simulink model "networked"  (Simulink 4.00)
settings: Solver=ode45  StartTime=0.0  StopTime=2  RelTol=1e-3
libraries: truetime x7
settings Model: Creator=anton  LastModifiedBy=anton  ExtModeAutoUpdateStatusClock=off

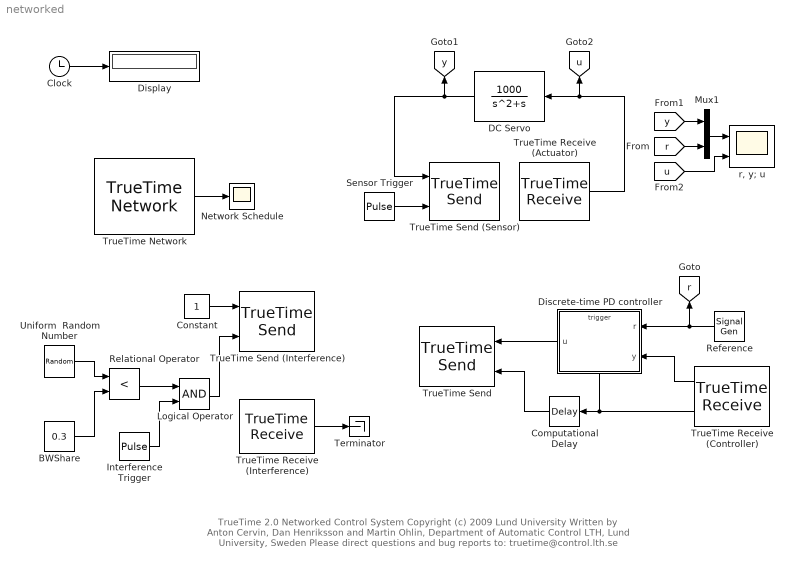
== system networked ==
  note: TrueTime 2.0  Networked Control System
      | Copyright (c) 2009 Lund University
      | Written by Anton Cervin, Dan Henriksson and Martin Ohlin,
      | Department of Automatic Control LTH, Lund University, Sweden
      | Please direct questions and bug reports to:  truetime@control.lth.se
  BWShare : Constant  Value=0.3
  Clock : Clock
      settings: DisplayTime=off  Decimation=10
  Computational Delay : TransportDelay  Orientation=left  DelayTime=0.002  InitialInput=0  BufferSize=1024  PadeOrder=0
  Constant : Constant  Value=1
  DC Servo : TransferFcn  Orientation=left  Numerator=[1000]  Denominator=[1 1 0]  AbsoluteTolerance=auto  Realization=auto
  Discrete-time PD controller : Subsystem  Orientation=left  TreatAsAtomicUnit=on  mask{K=1.0, Td=0.04, N=100, h=0.010}
      settings: RTWFcnNameOpts=Auto  RTWFileNameOpts=Auto
  Display : Display
      settings: Format=short
  Interference Trigger : DiscretePulseGenerator  PulseType=Time-based  Amplitude=1  Period=0.001  PulseWidth=50  PhaseDelay=0.006  SampleTime=1
  Logical Operator : Logic  Operator=AND  Inputs=2
  Mux1 : Mux  Inputs=2
  Network Schedule : Scope
      settings: TimeRange=2  YMin=1  YMax=3.5  SaveToWorkspace=off  SaveName=nschedule1  MaxDataPoints=5000
  Reference : SignalGenerator  Orientation=left  WaveForm=square  Amplitude=1  Frequency=1  Units=Hertz
  Relational Operator : RelationalOperator  Operator=<
  Sensor Trigger : DiscretePulseGenerator  PulseType=Time-based  Amplitude=1  Period=0.010  PulseWidth=50  PhaseDelay=0.006  SampleTime=1
  Terminator : Terminator
  TrueTime Network : truetime/TrueTime Network  AncestorBlock=truetime_MH/TrueTime Network  nwtype=CSMA/AMP (CAN)  nwnbr=1  nnodes=3  rate=80000  minsize=80  lossprob=0  seed=0  bandwidths=[0.5 0.25 0.25]  slotsize=80  schedule=[1 2 1 3]  memsize=80000  buftype=Common buffer  overflow=Retransmit  dynSchedule=0  miniSlotSize=0  NIT=0  QSortMode=FIFO  sync=0  irtSchedule=0  nrtLength=0  nodeGraph=0  scheduleoutput=on
  TrueTime Receive (Actuator) : truetime/TrueTime Receive  AncestorBlock=truetime_R12/TrueTime Receive  nwnbr=1  receiver=2  outdim=1  triggeroutput=off  senderoutput=off  lengthoutput=off  priorityoutput=off  timestampoutput=off  signalpoweroutput=off  msgIDoutput=off
  TrueTime Receive (Controller) : truetime/TrueTime Receive  Orientation=left  AncestorBlock=truetime_R12/TrueTime Receive  nwnbr=1  receiver=3  outdim=1  triggeroutput=on  senderoutput=off  lengthoutput=off  priorityoutput=off  timestampoutput=off  signalpoweroutput=off  msgIDoutput=off
  TrueTime Receive (Interference) : truetime/TrueTime Receive  AncestorBlock=truetime_R12/TrueTime Receive  nwnbr=1  receiver=1  outdim=1  triggeroutput=off  senderoutput=off  lengthoutput=off  priorityoutput=off  timestampoutput=off  signalpoweroutput=off  msgIDoutput=off
  TrueTime Send : truetime/TrueTime Send  Orientation=left  AncestorBlock=truetime_R12/TrueTime Send  trigger=either  nwnbr=1  sender=3  indim=1  recsource=internal  receiver=2  lengthsource=internal  length=80  priosource=internal  prio=3  msgIDsource=internal  msgID=0  dynamicSegment=dynamic
  TrueTime Send (Interference) : truetime/TrueTime Send  AncestorBlock=truetime_R12/TrueTime Send  trigger=rising  nwnbr=1  sender=1  indim=1  recsource=internal  receiver=1  lengthsource=internal  length=80  priosource=internal  prio=1  msgIDsource=internal  msgID=0  dynamicSegment=dynamic
  TrueTime Send (Sensor) : truetime/TrueTime Send  AncestorBlock=truetime_R12/TrueTime Send  trigger=rising  nwnbr=1  sender=2  indim=1  recsource=internal  receiver=3  lengthsource=internal  length=80  priosource=internal  prio=2  msgIDsource=internal  msgID=0  dynamicSegment=dynamic
  Uniform  Random Number : UniformRandomNumber  Minimum=0  Maximum=1  Seed=0  SampleTime=0.001
  "r, y; u" : Scope  NumInputPorts=2
      settings: TimeRange=2  YMin=-2~-3  YMax=2~3  SaveToWorkspace=off  SaveName=y  MaxDataPoints=5000
  tag scope: r=global, u=global, y=global
  wires:
  TrueTime Network/1 -> Network Schedule/1
  Mux1/1 -> "r, y; u"/1
  Clock/1 -> Display/1
  [r] -> Mux1/2
  [y] -> Mux1/1
  [u] -> "r, y; u"/2
  DC Servo/1 -> [y], TrueTime Send (Sensor)/1
  TrueTime Receive (Actuator)/1 -> DC Servo/1, [u]
  Sensor Trigger/1 -> TrueTime Send (Sensor)/2
  Constant/1 -> TrueTime Send (Interference)/1
  TrueTime Receive (Controller)/1 -> Discrete-time PD controller/2(y)
  TrueTime Receive (Controller)/2 -> Discrete-time PD controller/Trigger, Computational Delay/1
  Discrete-time PD controller/1(u) -> TrueTime Send/1
  Computational Delay/1 -> TrueTime Send/2
  Reference/1 -> Discrete-time PD controller/1(r), [r]
  TrueTime Receive (Interference)/1 -> Terminator/1
  Uniform  Random Number/1 -> Relational Operator/1
  BWShare/1 -> Relational Operator/2
  Relational Operator/1 -> Logical Operator/1
  Interference Trigger/1 -> Logical Operator/2
  Logical Operator/1 -> TrueTime Send (Interference)/2

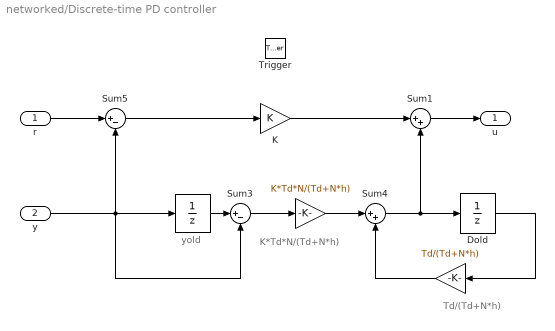
== system networked/Discrete-time PD controller ==
  note: yold
  note: Td/(Td+N*h)
  note: K*Td*N/(Td+N*h)
  r : Inport  Port=1  LatchInput=off
  y : Inport  Port=2  LatchInput=off
  Trigger : TriggerPort  TriggerType=either  OutputDataType=auto
  " " : UnitDelay  X0=0  SampleTime=-1
      settings: RTWStateStorageClass=Auto
  "             " : Gain  Gain=K*Td*N/(Td+N*h)  Multiplication=Element-wise(K.*u)  SaturateOnIntegerOverflow=on
  "              " : Gain  Orientation=left  Gain=Td/(Td+N*h)  Multiplication=Element-wise(K.*u)  SaturateOnIntegerOverflow=on
  Dold : UnitDelay  X0=0  SampleTime=-1
      settings: RTWStateStorageClass=Auto
  K : Gain  Gain=K  Multiplication=Element-wise(K.*u)  SaturateOnIntegerOverflow=on
  Sum1 : Sum  Inputs=|++  SaturateOnIntegerOverflow=on
  Sum3 : Sum  Inputs=|+-  SaturateOnIntegerOverflow=on
  Sum4 : Sum  Inputs=|++  SaturateOnIntegerOverflow=on
  Sum5 : Sum  Inputs=|+-  SaturateOnIntegerOverflow=on
  u : Outport  Port=1
  wires:
  Sum5/1 -> K/1
  "              "/1 -> Sum4/2
  " "/1 -> Sum3/1
  Sum4/1 -> Dold/1, Sum1/2
  Sum3/1 -> "             "/1
  "             "/1 -> Sum4/1
  Dold/1 -> "              "/1
  Sum1/1 -> u/1
  r/1 -> Sum5/1
  y/1 -> Sum5/2, " "/1, Sum3/2
  K/1 -> Sum1/1
